simulink model "full_model_arduino_final"  (R2020a)
settings: Solver=VariableStepAuto  StartTime=0.0  StopTime=ref(end,1)  RelTol=1e-3
values from neighbouring files (symbols this model uses):
  C = Ad.C    [Observer_mat.m]    (also in discretemodel.mat = [0  0  1  0; 0  0  0  1]; lqr_whitebox.m = sys.C; lqr_whitebox.mat = [0  0  1  0; 0  0  0  1]; matrices.mat = [0  0  1  0; 0  0  0  1])
  gamma = Ad.B    [Observer_mat.m]    (also in discretemodel.mat = [0.004353030085  4.48398112985e-06; 6.47055504813e-06  0.003; observer_matlab.m; observermatlab.m; observermatlab_final.m)
  h = tout(2)-tout(1)    [Linearize_whitebox.m]    (also in Linearize_whitebox_final.m; Observer_mat.m; lqr_whitebox.mat = 1.00037043897; matrices.mat = 1.00080032013)
  K = [0.871464143609  0.0262786205748; 0.0262786205748  0.871464143609; 0.341518856741  0.00295216925623; 0.00295216925623  0.341518856741]    [K_matrix.mat]    (also in K_matrix_final.mat = [0.107540648809  0.00297468629139; 0.00297468629139  0.10754; Observer_mat.m = place(phi.',C.',P).'; lqr_whitebox.m = lqr(A,B,Q,R); lqr_whitebox.mat = [9.8403850338  0.823629600444  7.09136571585  0.104667034235)
  L = lqr(A,B,Q,R)    [LQR.m]    (also in LQR_final.m; L_Lr_LQR.mat = [210.936834033  1.0429491506  82.9532479278  0.141237062686;; L_Lr_LQR_final.mat = [15.3959700225  0.0810970521206  45.9635678787  0.9358925165; L_Lr_Pole_Placement.mat = [382.498734136  0.681043508792  3740.11964319  0; 0.98277164)
  Lr = inv(Ldc)    [LQR.m]    (also in LQR_final.m; L_Lr_LQR.mat = [295.811652311  0.50314270449; -0.353029029898  433.02182351; L_Lr_LQR_final.mat = [63.2811082521  0.33594605992; -0.399513584683  63.309082518; L_Lr_Pole_Placement.mat = [4124.53994767  0; 0  5951.86777259])
  phi = Ad.A    [Observer_mat.m]    (also in discretemodel.mat = [0.991639753181 0.00295216925623 0.0399517774449 5.979211225; observer_matlab.m; observermatlab.m; observermatlab_final.m)
  u0 = [15; 15]    [observer_matlab.m]    (also in observermatlab_final.m)
  y0 = [300; 300]    [observer_matlab.m]    (also in observermatlab_final.m)
libraries: realtime_pacer_lib x1
settings Model: Creator=SIDTUDelft1  LastModifiedBy=SIDTUDelft1

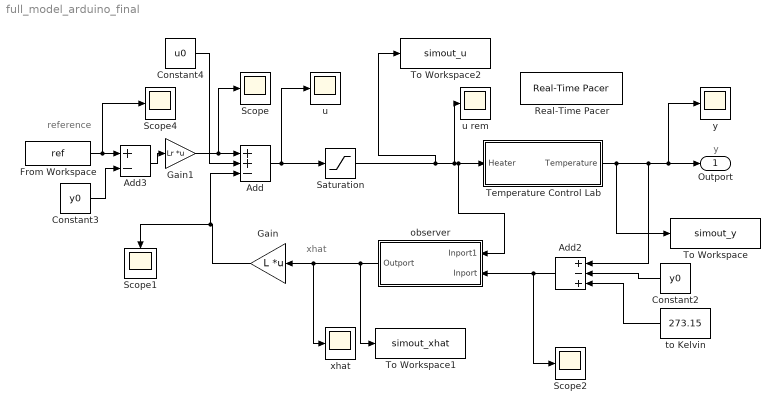
== system full_model_arduino_final ==
  note: reference
  note: xhat
  note: y
  Add : Sum  Inputs=++-  OutMin=[0]  OutMax=[100]
  Add2 : Sum  Inputs=+-+
  Add3 : Sum  Inputs=+-
  Constant2 : Constant  Value=y0
  Constant3 : Constant  Value=y0
  Constant4 : Constant  Value=u0  SampleTime=h
  From Workspace : FromWorkspace  VariableName=ref  SampleTime=h
  Gain : Gain  Gain=L  Multiplication=Matrix(K*u)
  Gain1 : Gain  Gain=Lr  Multiplication=Matrix(K*u)
  Real-Time Pacer : realtime_pacer_lib/Real-Time Pacer  simTimePerRealTime=h
  Saturation : Saturate  UpperLimit=100  LowerLimit=0
  Scope{,1..2,4} (4 alike) : Scope
  Temperature Control Lab : Subsystem
  To Workspace : ToWorkspace  VariableName=simout_y  SaveFormat=Timeseries  SampleTime=-1
  To Workspace1 : ToWorkspace  VariableName=simout_xhat  SaveFormat=Timeseries  SampleTime=-1
  To Workspace2 : ToWorkspace  VariableName=simout_u  SaveFormat=Timeseries  SampleTime=-1
  observer : Subsystem
  to Kelvin : Constant  Value=273.15
  u : Scope
  u rem : Scope
  xhat : Scope
  y : Scope
  Outport : Outport
  wires:
  observer/1(Outport) -> xhat/1, Gain/1, To Workspace1/1
  Saturation/1 -> To Workspace2/1, u rem/1, Temperature Control Lab/1(Heater), observer/1(Inport1)
  Constant2/1 -> Add2/2
  Add3/1 -> Gain1/1
  From Workspace/1 -> Scope4/1, Add3/1
  Constant3/1 -> Add3/2
  Add2/1 -> Scope2/1, observer/2(Inport)
  Temperature Control Lab/1(Temperature) -> To Workspace/1, Outport/1, y/1, Add2/1
  Add/1 -> Saturation/1, u/1
  Gain1/1 -> Scope/1, Add/1
  Gain/1 -> Add/3, Scope1/1
  Constant4/1 -> Add/2
  to Kelvin/1 -> Add2/3

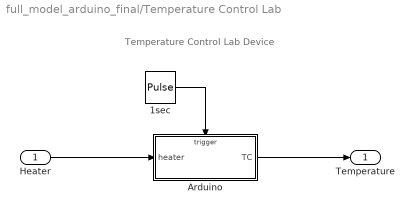
== system full_model_arduino_final/Temperature Control Lab ==
  note: Temperature Control Lab Device
  Heater : Inport
  1sec : DiscretePulseGenerator  PulseType=Time based  Period=1  PulseWidth=50
  Arduino : Subsystem  TreatAsAtomicUnit=on
  Temperature : Outport
  wires:
  1sec/1 -> Arduino/Trigger
  Arduino/1(TC) -> Temperature/1
  Heater/1 -> Arduino/1(heater)

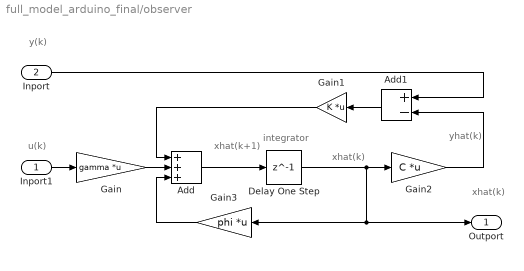
== system full_model_arduino_final/observer ==
  note: yhat(k)
  note: xhat(k+1)
  note: y(k)
  note: xhat(k)
  note: u(k)
  note: xhat(k)
  note: integrator
  Inport1 : Inport
  Inport : Inport  Port=2
  Add : Sum  Inputs=+++
  Add1 : Sum  Inputs=+-
  Delay One Step : Delay  DelayLength=1  SampleTime=h
  Gain : Gain  Gain=gamma  Multiplication=Matrix(K*u)
  Gain1 : Gain  Gain=K  Multiplication=Matrix(K*u)
  Gain2 : Gain  Gain=C  Multiplication=Matrix(K*u)
  Gain3 : Gain  Gain=phi  Multiplication=Matrix(K*u)
  Outport : Outport
  wires:
  Add/1 -> Delay One Step/1
  Add1/1 -> Gain1/1
  Gain1/1 -> Add/1
  Gain/1 -> Add/2
  Gain2/1 -> Add1/2
  Gain3/1 -> Add/3
  Inport/1 -> Add1/1
  Inport1/1 -> Gain/1
  Delay One Step/1 -> Gain3/1, Outport/1, Gain2/1

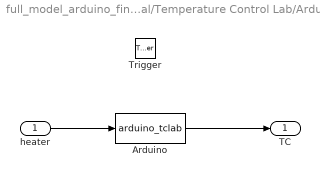
== system full_model_arduino_final/Temperature Control Lab/Arduino ==
  heater : Inport  LatchByDelayingOutsideSignal=on
  Trigger : TriggerPort  VariantControl=Variant
  Arduino : MATLABFcn  MATLABFcn=arduino_tclab
  TC : Outport  InitialOutput=23
  wires:
  heater/1 -> Arduino/1
  Arduino/1 -> TC/1
